simulink model "TEST_0_sim"  (R2014b)
settings: Solver=ode45  StartTime=0.0  StopTime=t_end  MaxStep=1  MinStep=1e-6  RelTol=1e-9  AbsTol=1e-9
values from neighbouring files (symbols this model uses):
  Mu = (3.9856e+14)    (= 398560000000000)    [ATV_laplace_potentials_test0.m]    (also in CW_anlytical.m; Controlled_motion_test1.m; EOS_test.m; Hill_TEST.m)
  R_0c = (R_0t+rand(3,1)*0.25*1e2)    [ATV_laplace_potentials_test0.m]    (also in CW_anlytical.m = [R_C;0;0]; Controlled_motion_test1.m = (R_0t+X_obs+rand(3,1)*0.25*1e2); Hill_TEST.m = (R_0t-rand(3,1)*0.5*1e2); Hill_TEST_INTEGR.m = (R_0t-[d_TC;0;0]))
  R_0t = [R_T;0;0]    [CW_anlytical.m]    (also in Controlled_motion_test1.m = [(r_Earth+h_orb);0;0]; EOS_test.m = [(r_Earth+h_orb);0;0]; Hill_TEST.m = [(r_Earth+h_orb);0;0]; Hill_TEST_INTEGR.m = [(r_Earth+h_orb);0;0])
  r_Earth = 6380*10^3    (= 6380000)    [ATV_laplace_potentials_test0.m]    (also in CW_anlytical.m; Controlled_motion_test1.m; EOS_test.m; Hill_TEST.m)
  V_0c = (V_0t+rand(3,1)*0.5*1e-1)    [ATV_laplace_potentials_test0.m]    (also in CW_anlytical.m = [0;sqrt(Mu/norm(R_0c));0]; Controlled_motion_test1.m = (V_0t-rand(3,1)*0.25*1e-2); Hill_TEST.m; Hill_TEST_INTEGR.m = [0;omega*R_C;0])
  V_0t = [0;sqrt(Mu/(r_Earth+h_orb));0]    [CW_anlytical.m]    (also in Controlled_motion_test1.m; EOS_test.m; Hill_TEST.m; Hill_TEST_INTEGR.m)
undefined symbols (not defined in the file or in its folder): r_0, v_0
libraries: vrlib x6
settings Model: Creator=peace  LastModifiedBy=peace

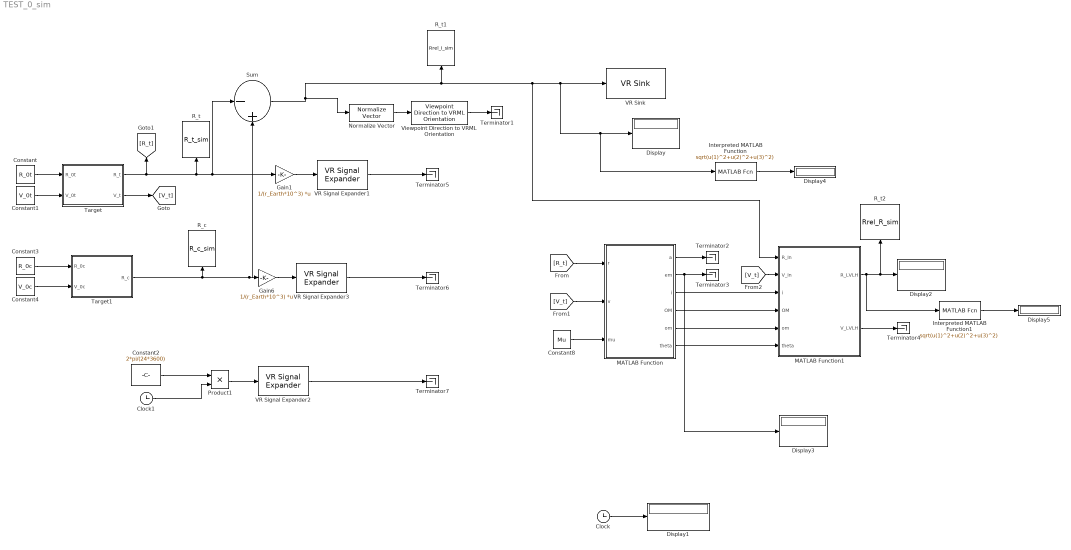
== system TEST_0_sim ==
  Clock : Clock
  Clock1 : Clock
  Constant : Constant  Value=R_0t  VectorParams1D=off
  Constant1 : Constant  Value=V_0t  VectorParams1D=off
  Constant2 : Constant  Value=2*pi/(24*3600)
  Constant3 : Constant  Value=R_0c  VectorParams1D=off
  Constant4 : Constant  Value=V_0c  VectorParams1D=off
  Constant8 : Constant  Value=Mu  VectorParams1D=off
  Display{,1..5} (6 alike) : Display
  Gain1 : Gain  Gain=1/(r_Earth*10^3)  Multiplication=Matrix(K*u)
  Gain6 : Gain  Gain=1/(r_Earth*10^3)  Multiplication=Matrix(K*u)
  Interpreted MATLAB Function : MATLABFcn  MATLABFcn=sqrt(u(1)^2+u(2)^2+u(3)^2)
  Interpreted MATLAB Function1 : MATLABFcn  MATLABFcn=sqrt(u(1)^2+u(2)^2+u(3)^2)
  MATLAB Function : MATLAB Function  TreatAsAtomicUnit=on
  MATLAB Function1 : MATLAB Function  TreatAsAtomicUnit=on
  Normalize Vector : vrlib/Utilities/Normalize Vector  maxzero=0
  Product1 : Product
  R_c : ToWorkspace  VariableName=R_c_sim  SaveFormat=Structure With Time  SampleTime=-1
  R_t : ToWorkspace  VariableName=R_t_sim  SaveFormat=Structure With Time  SampleTime=-1
  R_t1 : ToWorkspace  VariableName=Rrel_I_sim  SaveFormat=Structure With Time  SampleTime=-1
  R_t2 : ToWorkspace  VariableName=Rrel_R_sim  SaveFormat=Structure With Time  SampleTime=-1
  Sum : Sum  Inputs=|-+
  Target : Subsystem
  Target1 : Subsystem
  Terminator{1..7} (7 alike) : Terminator
  VR Signal Expander1 : vrlib/VR Signal Expander  outwidth=3  outidx=[1,2,3]
  VR Signal Expander2 : vrlib/VR Signal Expander  outwidth=4  outidx=[3]
  VR Signal Expander3 : vrlib/VR Signal Expander  outwidth=3  outidx=[1,2,3]
  VR Sink : vrlib/VR Sink  InstantiateOnLoad=on  SampleTime=0.1  ViewEnable=on  RemoteChange=off  RemoteView=off  FieldsWritten=Sphere.translation.3.1.1.double  WorldFileName=SS_SPH.wrl  AutoView=off  VideoDimensions=[]  AllowVariableSize=off
  Viewpoint Direction to VRML Orientation : vrlib/Utilities/Viewpoint Direction to VRML Orientation
  wires:
  Constant2/1 -> Product1/1
  Product1/1 -> VR Signal Expander2/1
  Clock1/1 -> Product1/2
  Target/1(R_t) -> [R_t], Sum/1, Gain1/1, R_t/1
  Constant/1 -> Target/1(R_0t)
  Constant1/1 -> Target/2(V_0t)
  VR Signal Expander3/1 -> Terminator6/1
  Target1/1(R_c) -> Sum/2, Gain6/1, R_c/1
  Constant3/1 -> Target1/1(R_0c)
  Constant4/1 -> Target1/2(V_0c)
  VR Signal Expander2/1 -> Terminator7/1
  Gain6/1 -> VR Signal Expander3/1
  VR Signal Expander1/1 -> Terminator5/1
  Gain1/1 -> VR Signal Expander1/1
  Sum/1 -> Normalize Vector/1, R_t1/1, MATLAB Function1/1(R_In), Interpreted MATLAB Function/1, Display/1, VR Sink/1
  Normalize Vector/1 -> Viewpoint Direction to VRML Orientation/1
  Viewpoint Direction to VRML Orientation/1 -> Terminator1/1
  Clock/1 -> Display1/1
  Target/2("V_t ") -> [V_t]
  [V_t] -> MATLAB Function/2(v)
  [R_t] -> MATLAB Function/1(r)
  Constant8/1 -> MATLAB Function/3(mu)
  MATLAB Function/1(a) -> Terminator2/1
  MATLAB Function/2(em) -> Display3/1, Terminator3/1
  MATLAB Function/3(i) -> MATLAB Function1/3(i)
  MATLAB Function/4(OM) -> MATLAB Function1/4(OM)
  MATLAB Function/5(om) -> MATLAB Function1/5(om)
  MATLAB Function/6(theta) -> MATLAB Function1/6(theta)
  MATLAB Function1/2(V_LVLH) -> Terminator4/1
  [V_t] -> MATLAB Function1/2(V_In)
  Interpreted MATLAB Function/1 -> Display4/1
  MATLAB Function1/1(R_LVLH) -> Interpreted MATLAB Function1/1, Display2/1, R_t2/1
  Interpreted MATLAB Function1/1 -> Display5/1

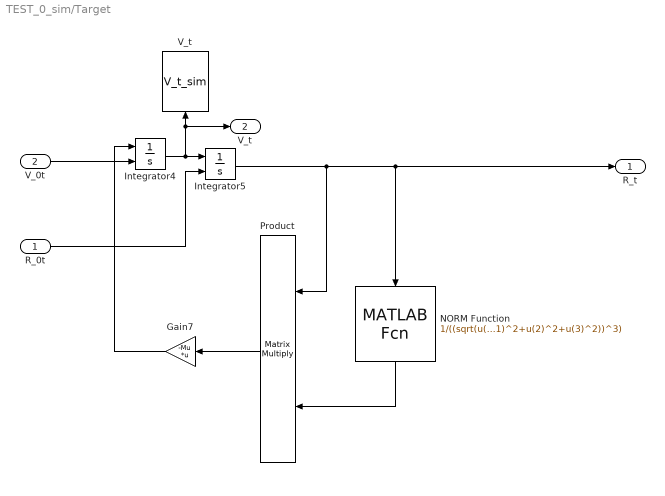
== system TEST_0_sim/Target ==
  R_0t : Inport
  V_0t : Inport  Port=2
  Gain7 : Gain  Gain=-Mu  Multiplication=Matrix(K*u)
  Integrator4 : Integrator  InitialConditionSource=external  InitialCondition=v_0
  Integrator5 : Integrator  InitialConditionSource=external  InitialCondition=r_0
  NORM Function : MATLABFcn  MATLABFcn=1/((sqrt(u(1)^2+u(2)^2+u(3)^2))^3)  OutputDimensions=1
  Product : Product  Multiplication=Matrix(*)
  V_t : ToWorkspace  VariableName=V_t_sim  SaveFormat=Structure With Time  SampleTime=-1
  R_t : Outport
  "V_t " : Outport  Port=2
  wires:
  Integrator5/1 -> R_t/1, NORM Function/1, Product/1
  Integrator4/1 -> Integrator5/1, "V_t "/1, V_t/1
  Gain7/1 -> Integrator4/1
  Product/1 -> Gain7/1
  NORM Function/1 -> Product/2
  V_0t/1 -> Integrator4/2
  R_0t/1 -> Integrator5/2

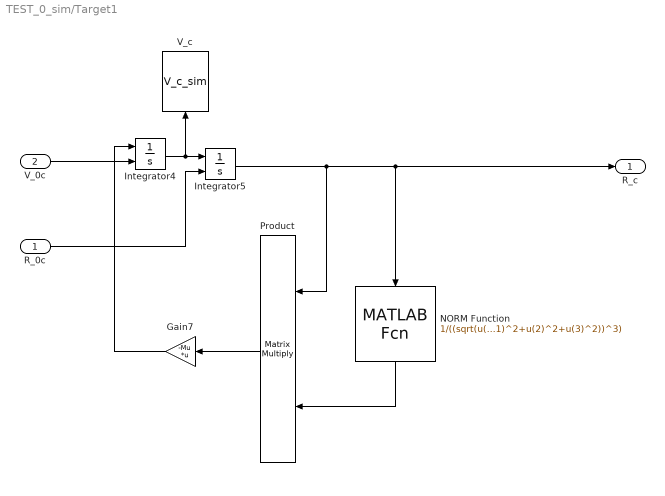
== system TEST_0_sim/Target1 ==
  R_0c : Inport
  V_0c : Inport  Port=2
  Gain7 : Gain  Gain=-Mu  Multiplication=Matrix(K*u)
  Integrator4 : Integrator  InitialConditionSource=external  InitialCondition=v_0
  Integrator5 : Integrator  InitialConditionSource=external  InitialCondition=r_0
  NORM Function : MATLABFcn  MATLABFcn=1/((sqrt(u(1)^2+u(2)^2+u(3)^2))^3)  OutputDimensions=1
  Product : Product  Multiplication=Matrix(*)
  V_c : ToWorkspace  VariableName=V_c_sim  SaveFormat=Structure With Time  SampleTime=-1
  R_c : Outport
  wires:
  Integrator5/1 -> R_c/1, NORM Function/1, Product/1
  Integrator4/1 -> Integrator5/1, V_c/1
  Gain7/1 -> Integrator4/1
  Product/1 -> Gain7/1
  NORM Function/1 -> Product/2
  V_0c/1 -> Integrator4/2
  R_0c/1 -> Integrator5/2

== matlab function TEST_0_sim/MATLAB Function1 ==
  data: R_In input; R_LVLH output; V_In input; i input; OM input; om input; theta input; V_LVLH output
function [R_LVLH,V_LVLH]=In2LVLH(R_In,V_In,i,OM,om,theta)

R_LVLH=zeros(3,1);
V_LVLH=zeros(3,1);


R_In=[R_In(1);R_In(2);R_In(3)];

ROT_Plane=[cos(om)*cos(OM)-sin(om)*cos(i)*sin(OM), -sin(om)*cos(OM)-cos(om)*cos(i)*sin(OM), sin(i)*sin(OM);
    cos(om)*sin(OM)+sin(om)*cos(i)*cos(OM), -sin(om)*sin(OM)+cos(om)*cos(i)*cos(OM), -sin(i)*cos(OM);
    sin(om)*sin(i), cos(om)*sin(i), cos(i)]; 

ROT_Theta=[cos(theta), sin(theta),  0;
          -sin(theta), cos(theta), 0;
             0       ,     0     ,1 ];
         
 

R_LVLH=ROT_Theta'* (ROT_Plane'* R_In);

hv=[0;0;0];
w=1;
%V_LVLH=V_In+w*cross(hv,R_LVLH);
V_LVLH=V_In;%NON E' VERO !!!!!
end

== matlab function TEST_0_sim/MATLAB Function ==
  data: r input; a output; v input; mu input; em output; i output; OM output; om output; theta output
function [a,em,i,OM,om,theta]=RV2OrbPar_My(r,v,mu)

rm=norm(r);
vm=norm(v);
a=mu/(((2*mu)/rm)-(vm^2));
h=cross(r,v);
hm=norm(h);
l=cross(v,h);
e=l/mu-r/rm;
em=norm(e);
i=acos(h(3)/hm);
kv=[0;0;1];
jv=[0;1;0];
iv=[1;0;0];

if norm(cross(kv,h))==0
n=iv;  
else
n=cross(kv,h)/norm(cross(kv,h));
end

    if dot(n,jv)>0
        OM=acos(dot(n,iv));
    else
        OM=2*pi-acos(dot(n,iv));
    end

if  abs(em) <1e-6
    
   om=0;
else
    
    if dot(e,kv)>0
        om=acos(dot(n,e)/em);
    else
        om=2*pi-acos(dot(n,e)/em);
    end
end

if em< 1e-6;

    theta=acos(dot(r/rm,iv));
    
else
    
    if dot(r,v)>0
        theta=acos(dot(r,e)/(rm*em));
    else
        theta=2*pi-acos(dot(r,e)/(rm*em));
    end
end

end
